simulink model "Demo"  (Simulink 10.1)
settings: Solver=FixedStepDiscrete  StartTime=0.0  StopTime=inf  FixedStep=0.001  RelTol=1e-3  EnableMultiTasking=on
libraries: arduinolib x9, simulink x1
settings Model: Creator=stum  LastModifiedBy=stum  ExtModeTrigDuration=2
settings DataIOCC: SaveFormat=Dataset  ReturnWorkspaceOutputs=on
settings OptimizationCC: EnhancedBackFolding=on  PassReuseOutputArgsAs=Individual arguments  ZeroExternalMemoryAtStartup=off  ZeroInternalMemoryAtStartup=off  LifeSpan=auto  MaxStackSize=64  OptimizeBlockOrder=speed  DifferentSizesBufferReuse=on  EfficientTunableParamExpr=on
settings DebuggingCC: UnderspecifiedInitializationDetection=Simplified  MergeDetectMultiDrivingBlocksExec=error  ParameterTunabilityLossMsg=error  SFUnexpectedBacktrackingDiag=error  SFNoUnconditionalDefaultTransitionDiag=error  SFExecutionAtInitializationDiag=warning
settings HardwareCC: ProdLargestAtomicInteger=Long  ProdLargestAtomicFloat=Double  ProdIntDivRoundTo=Zero  ProdEndianess=LittleEndian  ProdHWDeviceType=ARM Compatible->ARM Cortex
settings ModelReferenceCC: PropagateSignalLabelsOutOfModel=on
settings SFSimCC: SimUseLocalCustomCode=on  MATLABDynamicMemAlloc=off
settings RTWCC: Description=Embedded Coder  SystemTargetFile=ert.tlc  HardwareBoard=Arduino Due  TLCOptions=-aInlineSetEventsForThisBaseRateFcn=TLC_FALSE -aSuppressMultiTaskScheduler=TLC_FALSE -aRateBasedStepFcn=1  TemplateMakefile=ert_default_tmf  RTWUseLocalCustomCode=on  Toolchain=Arduino ARM  BuildConfiguration=Faster Runs
settings MATStruct: className=codertarget.tools.BuildHook  argsTopModelOnly=[]  excludedModels=[]  includeReferencedModels=on  includeTopModel=on  enabled=on  UseCoderTarget=[1.0]  TargetHardware=Arduino Due  RTOS=Baremetal  Scheduler_interrupt_source=[0.0]  DataVersion=2016.02  Baudrate=codertarget.arduinobase.registry.getBaudRate  COMPort=codertarget.arduinobase.internal.getExternalModeMexArgs('Serial')  Verbose=[0.0]  IPAddress=codertarget.arduinobase.internal.getExternalModeMexArgs('Ethernet')  Port=17725  Configuration=XCP on Serial  COMPortBaud=115200  signalBufferSize=[24576.0]  BuildAction=Build, load and run  DisableParallelBuild=[0.0]  Set_host_COM_port=Automatically  COM_port_number=/dev/tty.usbmodemfa131  Enable_SimulinkIO=[1.0]  Enable_overrun_detection=[0.0]  Digital_output_to_set_on_overrun=13  Analog_input_reference_voltage=[0.0]  Serial0_baud_rate=9600  Serial1_baud_rate=9600  Serial2_baud_rate=9600  Serial3_baud_rate=9600  I2C0BusSpeedHz=100000  I2C1BusSpeedHz=100000  SPI_clock_out_frequency=4000  SPI_mode=Mode 0 - Clock Polarity 0, Clock Phase 1  SPI_bitorder=MSB first  SDSlaveSelect=[4.0]  CANChipSelect=[10.0]  Disable_DHCP_Ethernet=[0.0]  Local_ip_address=192.168.0.20  Local_mac_address=DE:AD:BE:EF:FE:ED  Wifi_Hardware=WiFi shield  Disable_DHCP_Wifi=[0.0]  Wifi_ip_address=192.168.1.20  Wifi_SSID=yourNetwork  Set_Wifi_Encryption=None  Wifi_WEP_key=D0D0DEADF00DABBADEAFBEADED  Wifi_WEP_key_index=0  Wifi_WPA_password=secretPassword  Wifi_ESP8266_HW_serial_port=Serial 0  Enable_CustomServer=0  IP_address=184.106.153.149  CANBusSpeed=500  CANOscillatorFrequency=16  InterruptPin=[2.0]  AllowAllFilter=[0.0]  Buffer0IDType=Normal  AcceptanceMask0_Nor=0  AcceptanceFilter0_Nor=255  AcceptanceFilter1_Nor=255  AcceptanceMask0_Ext=0  AcceptanceFilter0_Ext=255  AcceptanceFilter1_Ext=255  Buffer1IDType=Normal  AcceptanceMask1_Nor=0  AcceptanceFilter2_Nor=255  AcceptanceFilter3_Nor=255  AcceptanceFilter4_Nor=255  AcceptanceFilter5_Nor=255  AcceptanceMask1_Ext=0  AcceptanceFilter2_Ext=255  AcceptanceFilter3_Ext=255  AcceptanceFilter4_Ext=255  AcceptanceFilter5_Ext=255
settings CodeAppCC: ForceParamTrailComments=on  IgnoreCustomStorageClasses=off  OperatorAnnotations=on  SimulinkDataObjDesc=on  SFDataObjDesc=on  InsertBlockDesc=on  StateflowObjectComments=off
settings ERTTargetCC: SupportContinuousTime=on  SupportVariableSizeSignals=on  ExtModeStaticAllocSize=24576
settings ConfigComp: CovMetricSettings=dwe  CovHtmlReporting=off  CovSaveCumulativeToWorkspaceVar=off  CovSaveSingleToWorkspaceVar=off  CovExternalEMLEnable=on

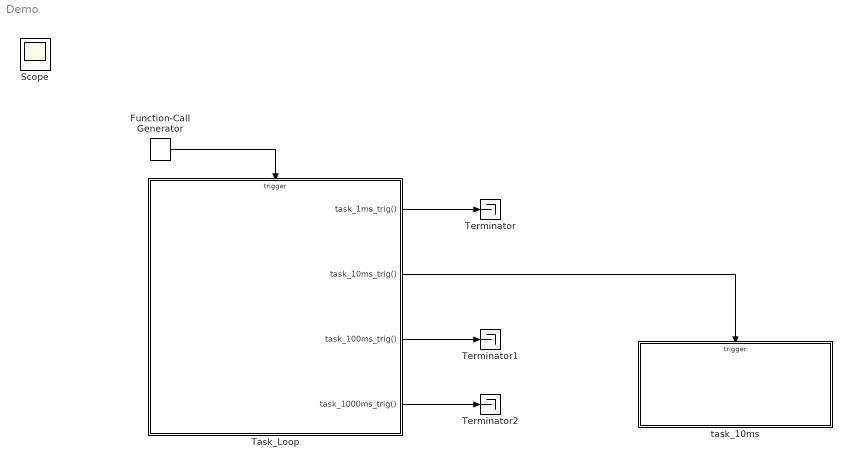
== system Demo ==
  Function-Call Generator : simulink/Ports & Subsystems/Function-Call Generator  sample_time=-1  numberOfIterations=1
  Task_Loop : Stateflow chart  TreatAsAtomicUnit=on
  Terminator : Terminator
  Terminator1 : Terminator
  Terminator2 : Terminator
  task_10ms : Subsystem  TreatAsAtomicUnit=on
  Scope : Scope
  wires:
  Function-Call Generator/1 -> Task_Loop/Trigger
  Task_Loop/2(task_10ms_trig()) -> task_10ms/Trigger
  Task_Loop/1(task_1ms_trig()) -> Terminator/1
  Task_Loop/3(task_100ms_trig()) -> Terminator1/1
  Task_Loop/4(task_1000ms_trig()) -> Terminator2/1

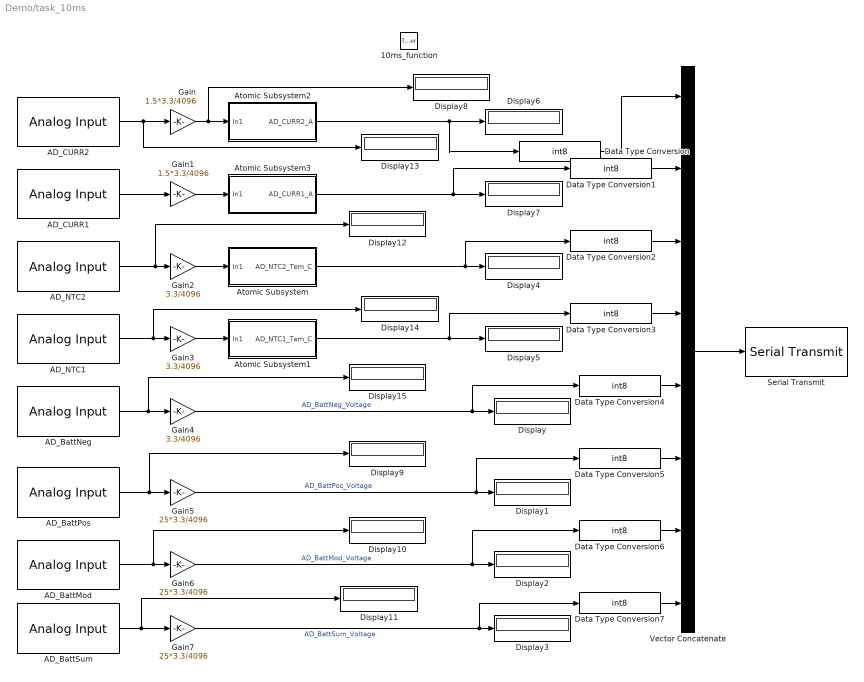
== system Demo/task_10ms ==
  10ms_function : TriggerPort  TriggerType=function-call  VariantControl=Variant
  AD_BattMod : arduinolib/Analog Input  pinNumber=1  ReadResultsOnly=off  ConversionTriggerSource=Software  ExternalTriggerType=uint32( 0 )  OutputDataType=uint16  EnableConversionCompleteNotify=off  EnableOuputStatus=off  SampleTime=-1  blockPlatform=arduino
  AD_BattNeg : arduinolib/Analog Input  pinNumber=3  ReadResultsOnly=off  ConversionTriggerSource=Software  ExternalTriggerType=uint32( 0 )  OutputDataType=uint16  EnableConversionCompleteNotify=off  EnableOuputStatus=off  SampleTime=-1  blockPlatform=arduino
  AD_BattPos : arduinolib/Analog Input  pinNumber=2  ReadResultsOnly=off  ConversionTriggerSource=Software  ExternalTriggerType=uint32( 0 )  OutputDataType=uint16  EnableConversionCompleteNotify=off  EnableOuputStatus=off  SampleTime=-1  blockPlatform=arduino
  AD_BattSum : arduinolib/Analog Input  pinNumber=0  ReadResultsOnly=off  ConversionTriggerSource=Software  ExternalTriggerType=uint32( 0 )  OutputDataType=uint16  EnableConversionCompleteNotify=off  EnableOuputStatus=off  SampleTime=-1  blockPlatform=arduino
  AD_CURR1 : arduinolib/Analog Input  pinNumber=6  ReadResultsOnly=off  ConversionTriggerSource=Software  ExternalTriggerType=uint32( 0 )  OutputDataType=uint16  EnableConversionCompleteNotify=off  EnableOuputStatus=off  SampleTime=-1  blockPlatform=arduino
  AD_CURR2 : arduinolib/Analog Input  pinNumber=7  ReadResultsOnly=off  ConversionTriggerSource=Software  ExternalTriggerType=uint32( 0 )  OutputDataType=uint16  EnableConversionCompleteNotify=off  EnableOuputStatus=off  SampleTime=-1  blockPlatform=arduino
  AD_NTC1 : arduinolib/Analog Input  pinNumber=4  ReadResultsOnly=off  ConversionTriggerSource=Software  ExternalTriggerType=uint32( 0 )  OutputDataType=uint16  EnableConversionCompleteNotify=off  EnableOuputStatus=off  SampleTime=-1  blockPlatform=arduino
  AD_NTC2 : arduinolib/Analog Input  pinNumber=5  ReadResultsOnly=off  ConversionTriggerSource=Software  ExternalTriggerType=uint32( 0 )  OutputDataType=uint16  EnableConversionCompleteNotify=off  EnableOuputStatus=off  SampleTime=-1  blockPlatform=arduino
  Atomic Subsystem : Subsystem  TreatAsAtomicUnit=on
  Atomic Subsystem1 : Subsystem  TreatAsAtomicUnit=on
  Atomic Subsystem2 : Subsystem  TreatAsAtomicUnit=on
  Atomic Subsystem3 : Subsystem  TreatAsAtomicUnit=on
  Data Type Conversion{,1..7} (8 alike) : DataTypeConversion  OutDataTypeStr=int8
  Display{,1..15} (16 alike) : Display
  Gain : Gain  Gain=1.5*3.3/4096
  Gain1 : Gain  Gain=1.5*3.3/4096
  Gain2 : Gain  Gain=3.3/4096
  Gain3 : Gain  Gain=3.3/4096
  Gain4 : Gain  Gain=3.3/4096
  Gain5 : Gain  Gain=25*3.3/4096
  Gain6 : Gain  Gain=25*3.3/4096
  Gain7 : Gain  Gain=25*3.3/4096
  Serial Transmit : arduinolib/Serial Transmit  portNumber=0  sendmode=println  label=data is  sendformat=Decimal  floatprecision=2  blockPlatform=arduino
  Vector Concatenate : Concatenate  NumInputs=8
  wires:
  AD_CURR2/1 -> Display13/1, Gain/1
  AD_CURR1/1 -> Gain1/1
  AD_NTC2/1 -> Display12/1, Gain2/1
  Gain2/1 -> Atomic Subsystem/1(In1)
  Gain3/1 -> Atomic Subsystem1/1(In1)
  AD_NTC1/1 -> Display14/1, Gain3/1
  AD_BattNeg/1 -> Display15/1, Gain4/1
  Gain4/1 -> Data Type Conversion4/1, Display/1  "AD_BattNeg_Voltage"
  Gain5/1 -> Data Type Conversion5/1, Display1/1  "AD_BattPos_Voltage"
  AD_BattPos/1 -> Display9/1, Gain5/1
  AD_BattMod/1 -> Display10/1, Gain6/1
  Gain6/1 -> Data Type Conversion6/1, Display2/1  "AD_BattMod_Voltage"
  Gain7/1 -> Data Type Conversion7/1, Display3/1  "AD_BattSum_Voltage"
  AD_BattSum/1 -> Display11/1, Gain7/1
  Atomic Subsystem/1(AD_NTC2_Tem_C) -> Data Type Conversion2/1, Display4/1
  Atomic Subsystem1/1(AD_NTC1_Tem_C) -> Data Type Conversion3/1, Display5/1
  Gain/1 -> Display8/1, Atomic Subsystem2/1(In1)
  Gain1/1 -> Atomic Subsystem3/1(In1)
  Atomic Subsystem2/1(AD_CURR2_A) -> Data Type Conversion/1, Display6/1
  Atomic Subsystem3/1(AD_CURR1_A) -> Data Type Conversion1/1, Display7/1
  Vector Concatenate/1 -> Serial Transmit/1
  Data Type Conversion/1 -> Vector Concatenate/1
  Data Type Conversion1/1 -> Vector Concatenate/2
  Data Type Conversion2/1 -> Vector Concatenate/3
  Data Type Conversion3/1 -> Vector Concatenate/4
  Data Type Conversion4/1 -> Vector Concatenate/5
  Data Type Conversion5/1 -> Vector Concatenate/6
  Data Type Conversion6/1 -> Vector Concatenate/7
  Data Type Conversion7/1 -> Vector Concatenate/8

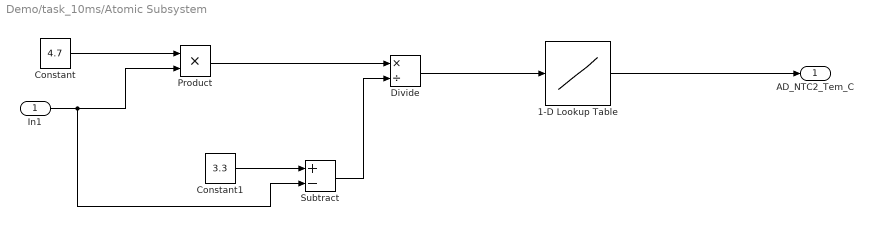
== system Demo/task_10ms/Atomic Subsystem ==
  In1 : Inport
  1-D Lookup Table : Lookup_n-D  NumberOfTableDimensions=1  BreakpointsForDimension1=[0.379900000000000 0.500200000000000 0.667600000000000 0.904000000000000 1.24310000000000 1.73800000000000 2.47340000000000 3.58820000000000 5.31460000000000 8.05120000000000 12.5005000000000 19.9380000000000 32.7547000000000]  BreakpointsForDimension1DataTypeStr=single  Table=[120 110 100 90 80 70 60 50 40 30 20 10 0]  TableDataTypeStr=single  InternalRulePriority=Speed  RndMeth=Simplest  InputSameDT=on
  Constant : Constant  Value=4.7  OutDataTypeStr=single
  Constant1 : Constant  Value=3.3  OutDataTypeStr=single
  Divide : Product  Inputs=*/
  Product : Product
  Subtract : Sum  Inputs=+-
  AD_NTC2_Tem_C : Outport
  wires:
  Constant/1 -> Product/1
  In1/1 -> Subtract/2, Product/2
  Product/1 -> Divide/1
  Divide/1 -> 1-D Lookup Table/1
  Subtract/1 -> Divide/2
  Constant1/1 -> Subtract/1
  1-D Lookup Table/1 -> AD_NTC2_Tem_C/1

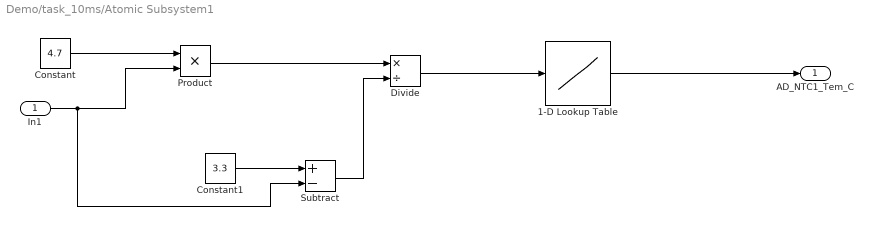
== system Demo/task_10ms/Atomic Subsystem1 ==
  In1 : Inport
  1-D Lookup Table : Lookup_n-D  NumberOfTableDimensions=1  BreakpointsForDimension1=[0.379900000000000 0.500200000000000 0.667600000000000 0.904000000000000 1.24310000000000 1.73800000000000 2.47340000000000 3.58820000000000 5.31460000000000 8.05120000000000 12.5005000000000 19.9380000000000 32.7547000000000]  BreakpointsForDimension1DataTypeStr=single  Table=[120 110 100 90 80 70 60 50 40 30 20 10 0]  TableDataTypeStr=single  InternalRulePriority=Speed  RndMeth=Simplest  InputSameDT=on
  Constant : Constant  Value=4.7  OutDataTypeStr=single
  Constant1 : Constant  Value=3.3  OutDataTypeStr=single
  Divide : Product  Inputs=*/
  Product : Product
  Subtract : Sum  Inputs=+-
  AD_NTC1_Tem_C : Outport
  wires:
  Constant/1 -> Product/1
  In1/1 -> Subtract/2, Product/2
  Product/1 -> Divide/1
  Divide/1 -> 1-D Lookup Table/1
  Subtract/1 -> Divide/2
  Constant1/1 -> Subtract/1
  1-D Lookup Table/1 -> AD_NTC1_Tem_C/1

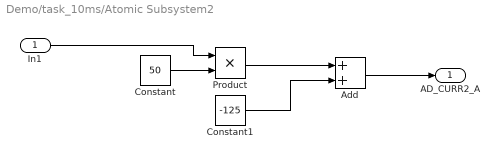
== system Demo/task_10ms/Atomic Subsystem2 ==
  In1 : Inport
  Add : Sum
  Constant : Constant  Value=50  OutDataTypeStr=single
  Constant1 : Constant  Value=-125  OutDataTypeStr=single
  Product : Product
  AD_CURR2_A : Outport
  wires:
  In1/1 -> Product/1
  Constant/1 -> Product/2
  Product/1 -> Add/1
  Constant1/1 -> Add/2
  Add/1 -> AD_CURR2_A/1

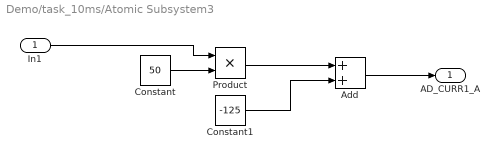
== system Demo/task_10ms/Atomic Subsystem3 ==
  In1 : Inport
  Add : Sum
  Constant : Constant  Value=50  OutDataTypeStr=single
  Constant1 : Constant  Value=-125  OutDataTypeStr=single
  Product : Product
  AD_CURR1_A : Outport
  wires:
  Add/1 -> AD_CURR1_A/1
  Constant1/1 -> Add/2
  Product/1 -> Add/1
  Constant/1 -> Product/2
  In1/1 -> Product/1

== stateflow chart Task_Loop ==
  settings: executeAtInitialization=1
  (default) -> (junction 12)
  (junction 12) -> (junction 13) : {task_tmr++;
      | task_10ms_tmr++;
      | task_100ms_tmr++;
      | task_1000ms_tmr++;
      | task_1ms_trig;}
  (junction 13) -> (junction 14) [order 1] : [task_10ms_tmr==10]
  (junction 13) -> (junction 15) [order 2]
  (junction 14) -> (junction 16) : {task_10ms_trig;
      | task_10ms_tmr=0;}
  (junction 16) -> (junction 15)
  (junction 15) -> (junction 17)
  (junction 17) -> (junction 18) [order 1] : [task_100ms_tmr==100]
  (junction 17) -> (junction 19) [order 2]
  (junction 18) -> (junction 20) : {task_100ms_trig;
      | task_100ms_tmr=0}
  (junction 20) -> (junction 19)
  (junction 19) -> (junction 21)
  (junction 21) -> (junction 22) [order 1] : [task_1000ms_tmr==1000]
  (junction 21) -> (junction 23) [order 2]
  (junction 22) -> (junction 24) : {task_1000ms_trig;
      | task_1000ms_tmr=0;}
  (junction 24) -> (junction 23)
  (junction 23) -> (junction 25)
  data: task_tmr local uint32 =0; task_10ms_tmr local uint32 =0; task_100ms_tmr local uint32 =0; task_1000ms_tmr local uint32 =0
  events: main_task input FUNCTION_CALL_EVENT; task_1ms_trig output FUNCTION_CALL_EVENT; task_10ms_trig output FUNCTION_CALL_EVENT; task_100ms_trig output FUNCTION_CALL_EVENT; task_1000ms_trig output FUNCTION_CALL_EVENT
